simulink model "Fig238"  (R2014a)
settings: Solver=ode45  StartTime=0.0  StopTime=10.0  RelTol=1e-3
undefined symbols (not defined in the file): TAU
libraries: commfilt2 x2
settings Model: Creator=Dennis Silage  LastModifiedBy=Silage
settings DataIOCC: SignalLoggingSaveFormat=ModelDataLogs
settings OptimizationCC: ExpressionDepthLimit=2147483647  InitFltsAndDblsToZero=on
settings DebuggingCC: UnderspecifiedInitializationDetection=Classic  FcnCallInpInsideContextMsg=UseLocalSettings  StateNameClashWarn=warning  StrictBusMsg=Warning
settings GRTTargetCC: CombineOutputUpdateFcns=off  GRTInterface=on

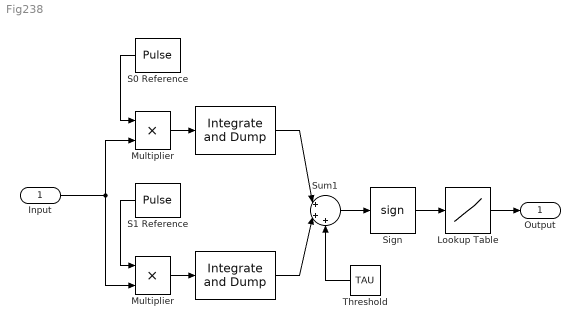
== system Fig238 ==
  Input : Inport
  " " : commfilt2/Integrate and Dump  obssamples=50  offsetsamples=0  nodump=off  roundingMode=Floor  overflowMode=off
  "  " : commfilt2/Integrate and Dump  obssamples=50  offsetsamples=0  nodump=off  roundingMode=Floor  overflowMode=off
  " Multiplier" : Product  RndMeth=Zero
  Lookup Table : Lookup  InputValues=[-1,0,1]  Table=[0,0,5]
  Multiplier : Product  RndMeth=Zero
  S0 Reference : DiscretePulseGenerator  PulseType=Time based  Period=1e-3  PulseWidth=98
  S1 Reference : DiscretePulseGenerator  PulseType=Time based  Period=1e-3  PulseWidth=98
  Sign : Signum
  Sum1 : Sum  Inputs=|+++
  Threshold : Constant  Value=TAU
  Output : Outport
  wires:
  Multiplier/1 -> " "/1
  S0 Reference/1 -> Multiplier/1
  " "/1 -> Sum1/1
  " Multiplier"/1 -> "  "/1
  S1 Reference/1 -> " Multiplier"/1
  Input/1 -> Multiplier/2, " Multiplier"/2
  Sign/1 -> Lookup Table/1
  Sum1/1 -> Sign/1
  Lookup Table/1 -> Output/1
  Threshold/1 -> Sum1/3
  "  "/1 -> Sum1/2
